simulink model "generator_model_2021"  (R2021b)
settings: Solver=ode45  StartTime=0.0  StopTime=2  FixedStep=1e-6  MaxStep=1e-6  RelTol=1e-5  EnableMultiTasking=on
InitFcn:
  | Rs=0.42;
  | Ls=0.96e-3;
  | C_phi=92.1952e-3;
  | poles=8;
  | Rload=15;
model workspace (MAT data in the model file):
  D = Simulink.Parameter
  D.Value = 0
  D.DataType = 'double'
  D.Complexity = 'real'
  D.Dimensions = [1 1]
  Power_previous = Simulink.Parameter
  Power_previous.Value = 0
  Power_previous.DataType = 'auto'
  Power_previous.Complexity = 'real'
  Power_previous.Dimensions = [1 1]
  R_eq = Simulink.Parameter
  R_eq.Value = 100
  R_eq.DataType = 'double'
  R_eq.Complexity = 'real'
  R_eq.Dimensions = [1 1]
  direction = Simulink.Parameter
  direction.Value = 0
  direction.DataType = 'auto'
  direction.Complexity = 'real'
  direction.Dimensions = [1 1]
libraries: spsDiodeLib x6, spsSeriesRLCBranchLib x6, spsControlledVoltageSourceLib x3, spsVoltageMeasurementLib x2, spsCurrentMeasurementLib x1, spsGroundLib x1, spsVariableCapacitorLib x1, spsVariableResistorLib x1, spspowerguiLib x1
settings Model: Creator=jwjansen  LastModifiedBy=maarten
settings DataIOCC: LimitDataPoints=on  SaveFormat=Array  ReturnWorkspaceOutputs=off
settings OptimizationCC: ExpressionDepthLimit=2147483647  LifeSpan=inf
settings DebuggingCC: UnderspecifiedInitializationDetection=Classic  MergeDetectMultiDrivingBlocksExec=none  SolverPrmCheckMsg=warning  FcnCallInpInsideContextMsg=warning  UnconnectedInputMsg=none  UnconnectedOutputMsg=none  UnconnectedLineMsg=none  StateNameClashWarn=warning  SFUnexpectedBacktrackingDiag=warning  SFNoUnconditionalDefaultTransitionDiag=warning  SFExecutionAtInitializationDiag=none  ArithmeticOperatorsInVariantConditions=warning
settings HardwareCC: ProdBitPerPointer=32  ProdBitPerSizeT=32  ProdBitPerPtrDiffT=32  ProdLargestAtomicFloat=None  ProdIntDivRoundTo=Undefined  ProdEndianess=Unspecified  ProdWordSize=32  ProdHWDeviceType=32-bit Generic
settings ModelReferenceCC: PropagateSignalLabelsOutOfModel=off
settings SFSimCC: SimUseLocalCustomCode=off  SimParseCustomCode=off  CustomCodeUndefinedFunction=UseInterfaceOnly
settings RTWCC: RTWUseLocalCustomCode=off  DLArmComputeVersion=20.02.1
settings CodeAppCC: StateflowObjectComments=on
settings GRTTargetCC: TargetLangStandard=C89/C90 (ANSI)  CombineOutputUpdateFcns=off  GRTInterface=on
settings ConfigComp: CovMetricSettings=dw  CovSaveCumulativeToWorkspaceVar=on  CovSaveSingleToWorkspaceVar=on  CovExternalEMLEnable=off
settings SimscapeCC: SimscapeNormalizeSystem=off

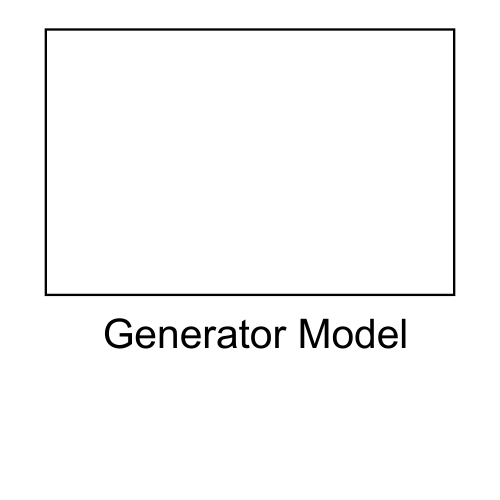
[thumbnail: Simulink's stored preview of the top-level diagram]
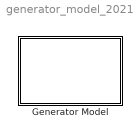
== system generator_model_2021 ==
  " Generator Model " : Subsystem

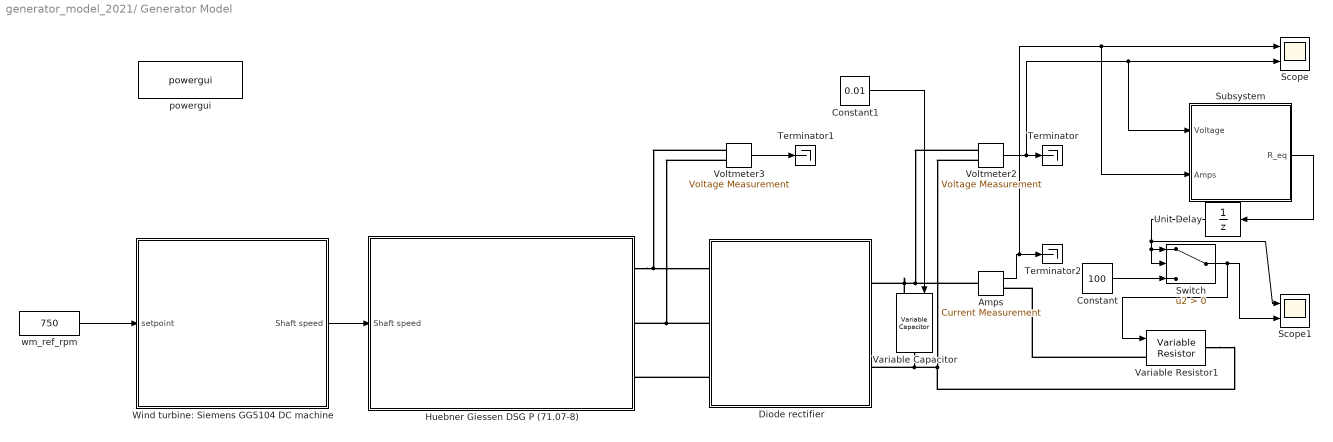
== system generator_model_2021/ Generator Model  ==
  Amps : spsCurrentMeasurementLib/Current Measurement  PhasorSimulation=off  OutputType=Complex  PSBequivalent=0
  Constant : Constant  Value=100
  Constant1 : Constant  Value=0.01
  Diode rectifier : Subsystem
  "Huebner Giessen DSG P (71.07-8) " : Subsystem
  Scope : Scope  NumInputPorts=2
  Scope1 : Scope  NumInputPorts=2
  Subsystem : Subsystem
  Switch : Switch  Criteria=u2 > Threshold
  Terminator : Terminator
  Terminator1 : Terminator
  Terminator2 : Terminator
  Unit Delay : UnitDelay  SampleTime=0.01  HasFrameUpgradeWarning=on
  Variable Capacitor : spsVariableCapacitorLib/Variable Capacitor  methode=Backward Euler  Cabsmin=1e-9  Initialize=off  vC0=0  C0=1e-6  iC0=0
  Variable Resistor1 : spsVariableResistorLib/Variable Resistor  Rabsmin=1
  Voltmeter2 : spsVoltageMeasurementLib/Voltage Measurement  PhasorSimulation=off  OutputType=Complex  PSBequivalent=0
  Voltmeter3 : spsVoltageMeasurementLib/Voltage Measurement  PhasorSimulation=off  OutputType=Complex  PSBequivalent=0
  "Wind turbine: Siemens GG5104 DC machine " : Subsystem
  powergui : spspowerguiLib/powergui  Priority=1  SimulationMode=Discrete  SampleTime=1e-5  frequency=60  Iterations=50  frequencyindice=0  Pbase=100e6  ErrMax=1e-4  UnitsV=kV  UnitsW=MW  buscounter=0  FunctionMessages=off  echomessages=off  EnableUseOfTLC=off  CurrentSourceSwitches=off  DisableSnubberDevices=off  DisableRonSwitches=off  DisableVfSwitches=off  DisplayEquations=off  AutomaticDiscreteSolvers=off  SolverType=Tustin  Interpol=off  ExternalGateDelay=off  methode=off  Ts=0  x0status=blocks  SPID=off  SwTol=0  HookPort=off  NonlinearTolerance=1e-4  nMaxIteration=100  ContinueOnMaxIteration=off  RestoreLinks=warning  ResistiveCurrentMeasurement=off  Frange=[0:2:500]  Ylog=off  Xlog=on  ShowGrid=off  save=off  variable=ZData  structure=0  ZoomFFT=off  StartTime=0.0  cycles=1  DisplayStyle=1  fundamental=60  FreqAxis=off  MaxFrequency=1000  frequencyindicesteady=1  RmsSteady=1  display=off
  wm_ref_rpm : Constant  Value=750
  wires:
  wm_ref_rpm/1 -> "Wind turbine: Siemens GG5104 DC machine "/1(setpoint)
  "Wind turbine: Siemens GG5104 DC machine "/1(Shaft speed) -> "Huebner Giessen DSG P (71.07-8) "/1(Shaft speed)
  Voltmeter3/1 -> Terminator1/1
  Amps/1 -> Subsystem/2(Amps), Scope/1, Terminator2/1
  Constant/1 -> Switch/3
  Voltmeter2/1 -> Scope/2, Subsystem/1(Voltage), Terminator/1
  Switch/1 -> Variable Resistor1/1, Scope1/2
  Subsystem/1(R_eq) -> Unit Delay/1
  Unit Delay/1 -> Switch/2, Switch/1, Scope1/1
  Constant1/1 -> Variable Capacitor/1
  connections:
  "Huebner Giessen DSG P (71.07-8) "/RConn1 -- Voltmeter3/LConn1 -- Diode rectifier/LConn1
  Diode rectifier/LConn2 -- Voltmeter3/LConn2 -- "Huebner Giessen DSG P (71.07-8) "/RConn2
  Diode rectifier/LConn3 -- "Huebner Giessen DSG P (71.07-8) "/RConn3
  Voltmeter2/LConn1 -- Amps/LConn1 -- Variable Capacitor/LConn1 -- Diode rectifier/RConn1
  Voltmeter2/LConn2 -- Variable Resistor1/RConn1 -- Variable Capacitor/RConn1 -- Diode rectifier/RConn2
  Variable Resistor1/LConn1 -- Amps/RConn1

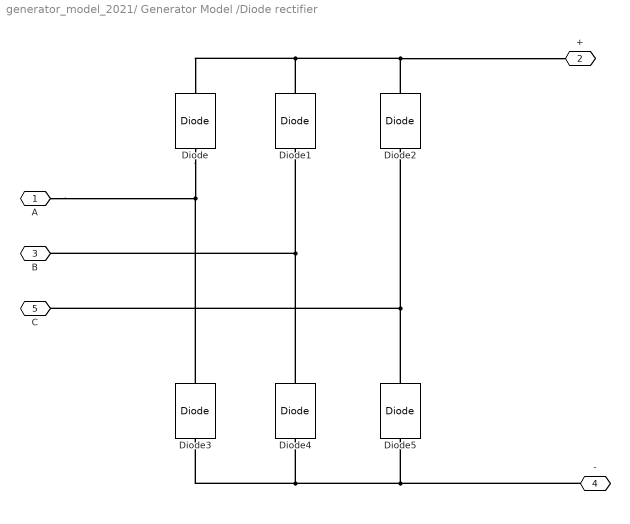
== system generator_model_2021/ Generator Model /Diode rectifier ==
  Diode{,1..5} (6 alike) : spsDiodeLib/Diode  Ron=0.01  Lon=0  Vf=0.85  IC=0  UseSnubber=off  Rs=500  Cs=250e-9  Measurements=off
  A : PMIOPort  Side=Left
  + : PMIOPort  Port=2  Side=Right
  B : PMIOPort  Port=3  Side=Left
  - : PMIOPort  Port=4  Side=Right
  C : PMIOPort  Port=5  Side=Left
  connections:
  Diode2/LConn1 -- C/RConn1 -- Diode5/RConn1
  +/RConn1 -- Diode2/RConn1 -- Diode1/RConn1 -- Diode/RConn1
  Diode3/LConn1 -- -/RConn1 -- Diode5/LConn1 -- Diode4/LConn1
  Diode3/RConn1 -- A/RConn1 -- Diode/LConn1
  Diode1/LConn1 -- B/RConn1 -- Diode4/RConn1

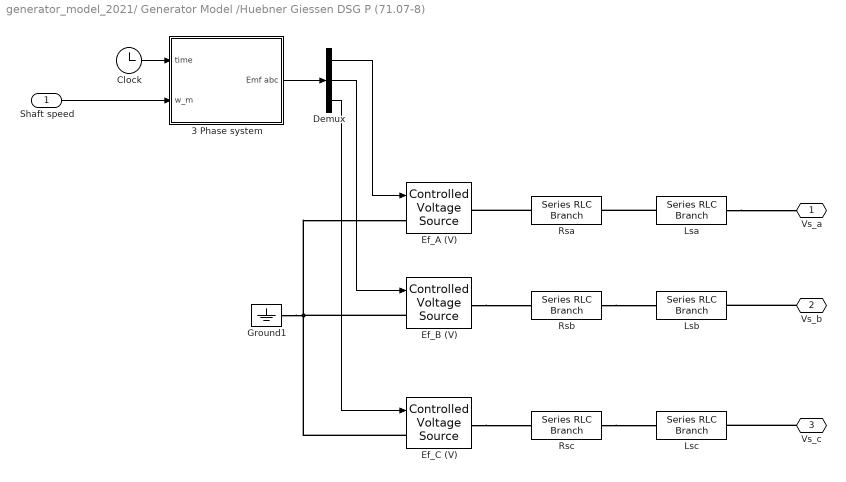
== system generator_model_2021/ Generator Model /Huebner Giessen DSG P (71.07-8)  ==
  Shaft speed : Inport
  "3 Phase system " : Subsystem
  Clock : Clock
  Demux : Demux  Outputs=3
  Ef_A (V) : spsControlledVoltageSourceLib/Controlled Voltage Source  Initialize=on  Source_Type=AC  Amplitude=0  Phase=0  Frequency=0  Measurements=None
  Ef_B (V) : spsControlledVoltageSourceLib/Controlled Voltage Source  Initialize=on  Source_Type=AC  Amplitude=0  Phase=0  Frequency=0  Measurements=None
  Ef_C (V) : spsControlledVoltageSourceLib/Controlled Voltage Source  Initialize=on  Source_Type=AC  Amplitude=0  Phase=0  Frequency=0  Measurements=None
  Ground1 : spsGroundLib/Ground  LConnTagsString=a
  Lsa : spsSeriesRLCBranchLib/Series RLC Branch  LConnTagsString=__new0  RConnTagsString=__new0  BranchType=L  Resistance=Rs  Inductance=Ls  SetiL0=off  InitialCurrent=0  Capacitance=1e-6  Setx0=off  InitialVoltage=0  Measurements=Branch current
  Lsb : spsSeriesRLCBranchLib/Series RLC Branch  LConnTagsString=__new0  RConnTagsString=__new0  BranchType=L  Resistance=Rs  Inductance=Ls  SetiL0=off  InitialCurrent=0  Capacitance=1e-6  Setx0=off  InitialVoltage=0  Measurements=Branch current
  Lsc : spsSeriesRLCBranchLib/Series RLC Branch  LConnTagsString=__new0  RConnTagsString=__new0  BranchType=L  Resistance=Rs  Inductance=Ls  SetiL0=on  InitialCurrent=0  Capacitance=1e-6  Setx0=off  InitialVoltage=0  Measurements=Branch current
  Rsa : spsSeriesRLCBranchLib/Series RLC Branch  LConnTagsString=__new0  RConnTagsString=__new0  BranchType=R  Resistance=Rs  Inductance=Ls  SetiL0=off  InitialCurrent=0  Capacitance=1e-6  Setx0=off  InitialVoltage=0  Measurements=Branch current
  Rsb : spsSeriesRLCBranchLib/Series RLC Branch  LConnTagsString=__new0  RConnTagsString=__new0  BranchType=R  Resistance=Rs  Inductance=Ls  SetiL0=off  InitialCurrent=0  Capacitance=1e-6  Setx0=off  InitialVoltage=0  Measurements=Branch current
  Rsc : spsSeriesRLCBranchLib/Series RLC Branch  LConnTagsString=__new0  RConnTagsString=__new0  BranchType=R  Resistance=Rs  Inductance=Ls  SetiL0=on  InitialCurrent=0  Capacitance=1e-6  Setx0=off  InitialVoltage=0  Measurements=Branch current
  Vs_a : PMIOPort  Side=Right
  Vs_b : PMIOPort  Port=2  Side=Right
  Vs_c : PMIOPort  Port=3  Side=Right
  wires:
  Demux/1 -> Ef_A (V)/1
  Demux/3 -> Ef_C (V)/1
  Demux/2 -> Ef_B (V)/1
  Shaft speed/1 -> "3 Phase system "/2(w_m)
  Clock/1 -> "3 Phase system "/1(time)
  "3 Phase system "/1("Emf abc ") -> Demux/1
  connections:
  Ef_B (V)/RConn1 -- Rsb/LConn1
  Lsa/RConn1 -- Vs_a/RConn1
  Vs_b/RConn1 -- Lsb/RConn1
  Ef_B (V)/LConn1 -- Ground1/LConn1 -- Ef_C (V)/LConn1 -- Ef_A (V)/LConn1
  Vs_c/RConn1 -- Lsc/RConn1
  Lsa/LConn1 -- Rsa/RConn1
  Ef_C (V)/RConn1 -- Rsc/LConn1
  Rsa/LConn1 -- Ef_A (V)/RConn1
  Rsb/RConn1 -- Lsb/LConn1
  Rsc/RConn1 -- Lsc/LConn1

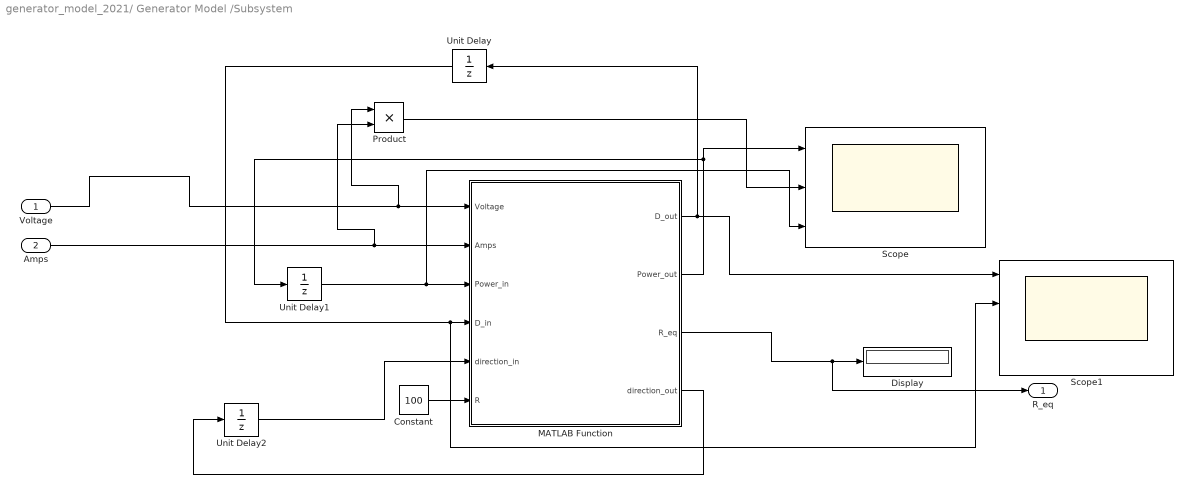
== system generator_model_2021/ Generator Model /Subsystem ==
  Voltage : Inport
  Amps : Inport  Port=2
  Constant : Constant  Value=100
  Display : Display
  MATLAB Function : MATLAB Function  TreatAsAtomicUnit=on  SystemSampleTime=0.01
  Product : Product
  Scope : Scope  NumInputPorts=3
  Scope1 : Scope  NumInputPorts=4
  Unit Delay : UnitDelay  InitialCondition=1  SampleTime=0.001  HasFrameUpgradeWarning=on
  Unit Delay1 : UnitDelay  SampleTime=0.001  HasFrameUpgradeWarning=on
  Unit Delay2 : UnitDelay  SampleTime=0.001  HasFrameUpgradeWarning=on
  R_eq : Outport
  wires:
  MATLAB Function/4(direction_out) -> Unit Delay2/1
  MATLAB Function/3(R_eq) -> R_eq/1, Display/1
  MATLAB Function/2(Power_out) -> Scope/1, Unit Delay1/1
  MATLAB Function/1(D_out) -> Unit Delay/1, Scope1/1
  Constant/1 -> MATLAB Function/6(R)
  Unit Delay1/1 -> Scope/3, MATLAB Function/3(Power_in)
  Unit Delay2/1 -> MATLAB Function/5(direction_in)
  Product/1 -> Scope/2
  Unit Delay/1 -> Scope1/2, MATLAB Function/4(D_in)
  Voltage/1 -> Product/1, MATLAB Function/1(Voltage)
  Amps/1 -> Product/2, MATLAB Function/2(Amps)

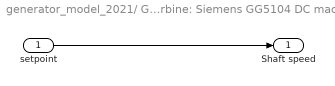
== system generator_model_2021/ Generator Model /Wind turbine: Siemens GG5104 DC machine  ==
  setpoint : Inport
  Shaft speed : Outport
  wires:
  setpoint/1 -> Shaft speed/1

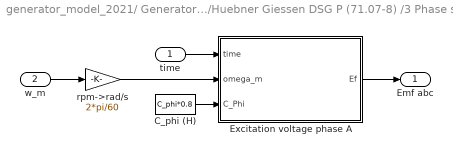
== system generator_model_2021/ Generator Model /Huebner Giessen DSG P (71.07-8) /3 Phase system  ==
  time : Inport
  w_m : Inport  Port=2
  C_phi (H) : Constant  Value=C_phi*0.8  VectorParams1D=off
  Excitation voltage phase A : Subsystem
  rpm->rad/s : Gain  Gain=2*pi/60
  "Emf abc " : Outport
  wires:
  w_m/1 -> rpm->rad/s/1
  C_phi (H)/1 -> Excitation voltage phase A/3(C_Phi)
  time/1 -> Excitation voltage phase A/1(time)
  rpm->rad/s/1 -> Excitation voltage phase A/2(omega_m)
  Excitation voltage phase A/1(Ef) -> "Emf abc "/1

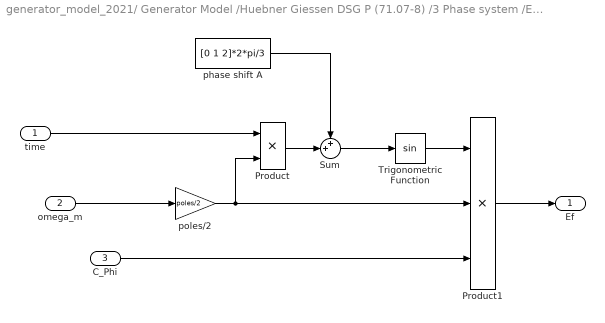
== system generator_model_2021/ Generator Model /Huebner Giessen DSG P (71.07-8) /3 Phase system /Excitation voltage phase A ==
  time : Inport
  omega_m : Inport  Port=2
  C_Phi : Inport  Port=3
  Product : Product  RndMeth=Zero
  Product1 : Product  Inputs=3  RndMeth=Zero
  Sum : Sum  Inputs=++|
  Trigonometric Function : Trigonometry
  phase shift A : Constant  Value=[0 1 2]*2*pi/3
  poles/2 : Gain  Gain=poles/2
  Ef : Outport
  wires:
  poles/2/1 -> Product/2, Product1/2
  Trigonometric Function/1 -> Product1/1
  phase shift A/1 -> Sum/1
  Product/1 -> Sum/2
  Product1/1 -> Ef/1
  C_Phi/1 -> Product1/3
  Sum/1 -> Trigonometric Function/1
  time/1 -> Product/1
  omega_m/1 -> poles/2/1

== matlab function generator_model_2021/ Generator Model /Subsystem/MATLAB Function ==
  settings: updateMethod=DISCRETE
  data: D_out output double [0..1]; Power_out output double; Voltage input double; Amps input double; R_eq output double; Power_in input double; D_in input double [0..1]; direction_in input double; R input double; direction_out output double
function [D_out, Power_out, R_eq, direction_out] = fcn(Voltage, Amps, Power_in, D_in, direction_in, R)

Power = Voltage * Amps;

if Power < Power_in
    if direction_in == 1
        direction = 0;
    else
        direction = 1;
    end
    %direction = ~direction_in;
else 
    direction = direction_in;
end

D = D_in + (0.01 * direction) - (0.01 * (1 - direction));

R_eq = D^2 * R;
Power_out = Power;
D_out = D;
direction_out = direction;
